simulink model "sideslip_loop"  (R2014b)
settings: Solver=ode45  StartTime=0.0  StopTime=10.0  MaxStep=0.1  RelTol=1e-3
values from neighbouring files (symbols this model uses):
  a_beta_1 = -P.rho*Va*P.S_wing/(2*P.mass) * P.C_Y_beta    [tuning.m]
  a_beta_2 = P.rho*Va*P.S_wing/(2*P.mass) * P.C_Y_delta_r    [tuning.m]
  k_i_beta = (1/a_beta_2) * ((a_beta_1 + a_beta_2*k_p_beta)/(2*zeta_beta))^2    [tuning.m]
  k_p_beta = delta_r_max/e_beta_max * sign(a_beta_2)    [tuning.m]
settings Model: Creator=kunalmenda  LastModifiedBy=kunalmenda

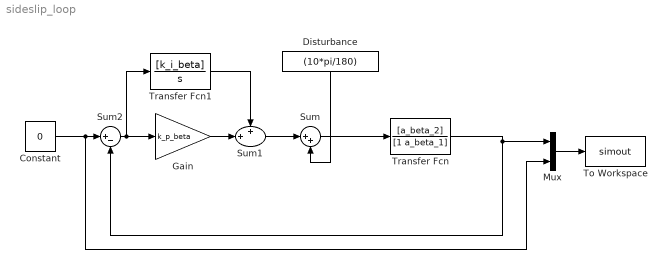
== system sideslip_loop ==
  Constant : Constant  Value=0
  Disturbance : Constant  Value=(10*pi/180)
  Gain : Gain  Gain=k_p_beta
  Mux : Mux  Inputs=2
  Sum : Sum  Inputs=|++
  Sum1 : Sum  Inputs=++|
  Sum2 : Sum  Inputs=|+-
  To Workspace : ToWorkspace  VariableName=simout  SaveFormat=Timeseries  SampleTime=-1
  Transfer Fcn : TransferFcn  Numerator=[a_beta_2]  Denominator=[1 a_beta_1]
  Transfer Fcn1 : TransferFcn  Numerator=[k_i_beta]  Denominator=[1 0]
  wires:
  Sum2/1 -> Transfer Fcn1/1, Gain/1
  Disturbance/1 -> Sum/2
  Transfer Fcn/1 -> Mux/1, Sum2/2
  Constant/1 -> Mux/2, Sum2/1
  Mux/1 -> To Workspace/1
  Sum1/1 -> Sum/1
  Sum/1 -> Transfer Fcn/1
  Transfer Fcn1/1 -> Sum1/1
  Gain/1 -> Sum1/2
